simulink model "Rod_end_v7c"  (R2023a)
settings: Solver=ode1be  StartTime=0.0  StopTime=3  FixedStep=1e-6  MaxStep=1e-5  RelTol=1e-3
values from neighbouring files (symbols this model uses):
  A1_la = 5.710000e-003    (= 0.00571)    [C1_Actuator_1_Data.m]
  A2_la = 5.710000e-003    (= 0.00571)    [C1_Actuator_1_Data.m]
  a_jetpipe_area = 0    [B2_Main_file_Double_Active_Standby_System.m]
  A_svfb = 79.12.*1E-9.*sqrt(pi)    [B2_Main_file_Double_Active_Standby_System.m]
  a_svfb0_1 = 1E-3    (= 0.001)    [B2_Main_file_Double_Active_Standby_System.m]
  a_svfb0_2 = 0    [B2_Main_file_Double_Active_Standby_System.m]
  Afl_sv = dfl_sv^2*pi/4    (= 2.01519637574e-09)    [C1_Actuator_1_Data.m]
  Ag_sv = 18e-6    (= 1.8e-05)    [C1_Actuator_1_Data.m]
  air_gap0_1 = 0    [B2_Main_file_Double_Active_Standby_System.m]
  air_gap_fault_time = 10000    [B2_Main_file_Double_Active_Standby_System.m]
  Alpha_p0 = eta-acos((L^2+t^2-s^2)/(2*L*t))    [Parametri_rod_end.m]
  Asp_sv = 1.35e-5    (= 1.35e-05)    [C1_Actuator_1_Data.m]
  B0_sv = 0.460    (= 0.46)    [C1_Actuator_1_Data.m]
  b_airgap = 0.3    [B2_Main_file_Double_Active_Standby_System.m]
  b_fbspring = 2E-3    (= 0.002)    [B2_Main_file_Double_Active_Standby_System.m]
  b_max = 0*0.0001    (= 0)    [C1_Actuator_1_Data.m]
  beta = 800000000    [D4_Fluid.m]    (also in Rapporto_di_trasmissione.m = acos((L-t.*cos(alpha))./s))
  Beta0 = acos((L-t*cos(Alpha0))/s)    [Parametri_rod_end.m]
  beta_LVDT = 0    [aggiunte.m]
  bf_sv = 0.45    [C1_Actuator_1_Data.m]
  bsp_sv = 0.25    [C1_Actuator_1_Data.m]
  c = 55    [Parametri_rod_end.m]
  C_svfb = 1    [B2_Main_file_Double_Active_Standby_System.m]
  Cdmax_sv = 0.7392    [C1_Actuator_1_Data.m]
  Cdmin_sv = 0.6428    [C1_Actuator_1_Data.m]
  CLa = 900000    [aggiunte.m]
  Csa_la = 0.02*sqrt(Ksa_la*Meq_la)    [C1_Actuator_1_Data.m]
  Damping = 1e3    (= 1000)    [Parametri_rod_end.m]
  Damping_rot = 100    [Parametri_rod_end.m]
  Del_on = 1    [B2_Main_file_Double_Active_Standby_System.m]
  demag0_1 = 0    [B2_Main_file_Double_Active_Standby_System.m]
  dfl_sv = 5.0654e-5    (= 5.0654e-05)    [C1_Actuator_1_Data.m]
  dt_sim = 1e-5    (= 1e-05)    [B2_Main_file_Double_Active_Standby_System.m]
  enable_jetpipe_distorsion = 0    [B2_Main_file_Double_Active_Standby_System.m]
  eta = deg2rad(15)    [Parametri_rod_end.m]
  F_att_sv = 4    [C1_Actuator_1_Data.m]
  FH = FH+0.175*pi*Dd_se(ii)*(-0.884+0.0206*Hs_se(ii)-0.0001*(Hs_se(ii))^2)*Tw_se(ii)    [D2_Data_seal.m]
  first_cycle = 0    [B2_Main_file_Double_Active_Standby_System.m]
  flight_hours = 8    [B2_Main_file_Double_Active_Standby_System.m]
  g = 9.81    [Parametri_rod_end.m]
  g_sv = G_sv/l0_sv    (= 0)    [C1_Actuator_1_Data.m]
  Gamma_la = 1.667e4    (= 16670)    [C1_Actuator_1_Data.m]
  gap_ms = 0    [C1_Actuator_1_Data.m]
  Gq_sv = 0.069    [C1_Actuator_1_Data.m]
  Gust_stiffness_jetpipe = 1e8    (= 100000000)    [B2_Main_file_Double_Active_Standby_System.m]
  Gust_threshold = 10000    [B2_Main_file_Double_Active_Standby_System.m]
  h_fbspring = 1E-3    (= 0.001)    [B2_Main_file_Double_Active_Standby_System.m]
  h_sv = H_sv/l0_sv    (= 0)    [C1_Actuator_1_Data.m]
  hr_sv = 6e-6    (= 6e-06)    [C1_Actuator_1_Data.m]
  hyd_fluid_repl = 20    [B2_Main_file_Double_Active_Standby_System.m]
  I = 2.3    [Parametri_rod_end.m]    (also in Rapporto_di_trasmissione.m)
  imax_sv = 8e-3    (= 0.008)    [C1_Actuator_1_Data.m]
  Initial_condition = [0;0;0.000]    [Parametri_rod_end.m]
  Ixx_out = 0.0000321    (= 3.21e-05)    [Parametri_rod_end.m]
  Iyy_in = 0.0000008    (= 8e-07)    [Parametri_rod_end.m]
  Iyy_out = 0.0000035    (= 3.5e-06)    [Parametri_rod_end.m]
  Izz_in = 0.00000011    (= 1.1e-07)    [Parametri_rod_end.m]
  Izz_out = 0.0000337    (= 3.37e-05)    [Parametri_rod_end.m]
  Ja_sv = 1.0575e-5    (= 1.0575e-05)    [C1_Actuator_1_Data.m]
  jetpipe_initialpos = 0    [B2_Main_file_Double_Active_Standby_System.m]
  jetpipe_passage_area = 1    [B2_Main_file_Double_Active_Standby_System.m]
  k = 4/(3*pi*(sigma_j+sigma_k))*((R_in*R_out)/(R_in+R_out))^0.5    (= 15092124693.8)    [Parametri_rod_end.m]
  k_airgap = 0.5/100*0.01    (= 5e-05)    [B2_Main_file_Double_Active_Standby_System.m]
  k_c0_jetpipe_area = 0*1e-1    (= 0)    [B2_Main_file_Double_Active_Standby_System.m]
  k_sv = mup_sv*Vp_sv/(2*B0_sv*l0_sv)-1    (= 16.0383594613)    [C1_Actuator_1_Data.m]
  Kf_sv = 301.6    [C1_Actuator_1_Data.m]
  KFPi = zeros(m,1)    [D2_Data_seal.m]
  Kli1 = 0    [C1_Actuator_1_Data.m]
  Kli2 = 0    [C1_Actuator_1_Data.m]
  Ksa_la = 12480000    [C1_Actuator_1_Data.m]
  Kw_sv = 14.5    [C1_Actuator_1_Data.m]
  L = 0.37    [Parametri_rod_end.m]    (also in Rapporto_di_trasmissione.m = l+delta_l)
  l0_sv = 0.5e-3    (= 0.0005)    [C1_Actuator_1_Data.m]
  L_c = imax_sv    (= 0.008)    [C1_Actuator_1_Data.m]
  L_la1 = 0.059900    (= 0.0599)    [C1_Actuator_1_Data.m]
  L_la2 = 0.084800    (= 0.0848)    [C1_Actuator_1_Data.m]
  la_sv = 41e-3    (= 0.041)    [C1_Actuator_1_Data.m]
  lambda_LVDT = 0*0.005*1.5    (= 0)    [aggiunte.m]
  lf = 0.025    [C1_Actuator_1_Data.m]    (also in C2_Actuator_2_Data.m)
  LVDTsize0 = 1    [aggiunte.m]
  m_in = 0.0215    [Parametri_rod_end.m]
  m_out = 0.1    [Parametri_rod_end.m]
  m_thermal = 0    [B2_Main_file_Double_Active_Standby_System.m]
  Mcyl_la = 30.425550    (= 30.42555)    [C1_Actuator_1_Data.m]
  Mrod_la = 11.313490    (= 11.31349)    [C1_Actuator_1_Data.m]
  msp_sv = 0.005    [C1_Actuator_1_Data.m]
  mua_sv = 4*pi/1e7    (= 1.25663706144e-06)    [C1_Actuator_1_Data.m]
  mup_sv = 1.1*4*pi/1e7    (= 1.38230076758e-06)    [C1_Actuator_1_Data.m]
  n1_sv = 1140    [C1_Actuator_1_Data.m]
  n2_sv = 1140    [C1_Actuator_1_Data.m]
  n_svfb = 3    [B2_Main_file_Double_Active_Standby_System.m]
  null_shift = -1+2*rand(1,1)    [B2_Main_file_Double_Active_Standby_System.m]
  null_shift_sign = -1+((-1+2*rand(1,1))>=0)*2    [B2_Main_file_Double_Active_Standby_System.m]
  OV_R1 = 0*2.344e-05    (= 0)    [C1_Actuator_1_Data.m]
  OV_R2 = 0*2.344e-05    (= 0)    [C1_Actuator_1_Data.m]
  OV_S1 = 0*2.344e-05    (= 0)    [C1_Actuator_1_Data.m]
  OV_S2 = 0*2.344e-05    (= 0)    [C1_Actuator_1_Data.m]
  P01_la = Pmean-DP_eq    [C1_Actuator_1_Data.m]
  P02_la = Pmean+DP_eq    [C1_Actuator_1_Data.m]
  perc_passage_area0_1 = 0    [B2_Main_file_Double_Active_Standby_System.m]
  Pocl_A = 0    [C1_Actuator_1_Data.m]
  Pocl_B = 0    [C1_Actuator_1_Data.m]
  Pr = 600000    [B2_Main_file_Double_Active_Standby_System.m]
  Ps = 35000000    [B2_Main_file_Double_Active_Standby_System.m]
  R_in = 0.019    [Parametri_rod_end.m]
  R_out = 0.0195    [Parametri_rod_end.m]
  R_th1 = 0    [B2_Main_file_Double_Active_Standby_System.m]
  Remax_sv = 5000    [C1_Actuator_1_Data.m]
  Resistance = 1    [C1_Actuator_1_Data.m]
  rj_sv = 1e-6    (= 1e-06)    [C1_Actuator_1_Data.m]
  Rp02_svspring = 1014    [B2_Main_file_Double_Active_Standby_System.m]
  s = 0.11    [Parametri_rod_end.m]    (also in Rapporto_di_trasmissione.m)
  sigma_0LVDT = 0*0.01*1.5*5    (= 0)    [aggiunte.m]
  ST_AD = ceil(10000/fs_AD)/10000    [C1_Actuator_1_Data.m]
  Stiffness_rot = 1e3    (= 1000)    [Parametri_rod_end.m]
  Stifness = 1e8    (= 100000000)    [Parametri_rod_end.m]
  sv_crackON1 = 0    [B2_Main_file_Double_Active_Standby_System.m]
  sv_crackON2 = 0    [B2_Main_file_Double_Active_Standby_System.m]
  T0 = 0    [aggiunte.m]
  tau_w1 = 0    [B2_Main_file_Double_Active_Standby_System.m]
  ... (+14 more)
undefined symbols (not defined in the file or in its folder): Ixx_in, magnitude, mass, muu, Newton, R_sp_C, Raphson
libraries: simulink x16, matrix_library x12, sharedutil x2
(part 2 of 4)

== system Rod_end_v7c/Crank position/Moment ==
  M_ext : Inport
  F_ms : Inport  Port=2
  Beta : Inport  Port=3
  Alpha_p : Inport  Port=4
  Constant : Constant  Value=s
  Cos : Trigonometry  Operator=cos
  Demux : Demux  Outputs=3
  Product : Product
  Product1 : Product
  Product2 : Product
  Scope : Scope
  Sin : Trigonometry
  Subtract : Sum  Inputs=+-
  Sum : Sum
  Sum2 : Sum
  Terminator : Terminator
  M : Outport
  wires:
  Beta/1 -> Sum2/2
  Demux/1 -> Product/2
  Product/1 -> Sum/1
  Sum2/1 -> Sin/1, Cos/1
  Sum/1 -> Scope/1, Product2/2
  F_ms/1 -> Demux/1
  Product1/1 -> Sum/2
  Sin/1 -> Product/1
  Constant/1 -> Product2/1
  Demux/3 -> Terminator/1
  Cos/1 -> Product1/1
  Alpha_p/1 -> Sum2/1
  Demux/2 -> Product1/2
  Product2/1 -> Subtract/1
  Subtract/1 -> M/1
  M_ext/1 -> Subtract/2

== system Rod_end_v7c/Crank position/Rot_equilibrium ==
  note: theta_dd
  note: theta_d
  M : Inport
  M_ext : Inport  Port=2
  Angle : Inport  Port=3
  Demux : Demux  Outputs=3
  Gain : Gain  Gain=mass*g*s/3
  Gain1 : Gain  Gain=c
  Gain2 : Gain  Gain=1/I
  Integrator : Integrator
  Integrator1 : Integrator
  Sin : Trigonometry
  Sum1 : Sum  Inputs=++--
  Terminator : Terminator
  Terminator1 : Terminator
  Theta : Outport
  Theta_d : Outport  Port=2
  wires:
  Angle/1 -> Sin/1
  Sum1/1 -> Gain2/1
  Gain1/1 -> Sum1/4
  Gain2/1 -> Integrator/1
  Integrator/1 -> Integrator1/1, Theta_d/1, Gain1/1
  Gain/1 -> Sum1/3
  M/1 -> Sum1/1
  Integrator1/1 -> Theta/1
  Demux/3 -> Sum1/2
  Sin/1 -> Gain/1
  M_ext/1 -> Demux/1
  Demux/2 -> Terminator/1
  Demux/1 -> Terminator1/1

== system Rod_end_v7c/Crank position/Trigonometry for V_sup ==
  Theta_d : Inport
  Sin : Inport  Port=2
  Cos : Inport  Port=3
  Constant13 : Constant  Value=s
  Constant14 : Constant  Value=0
  Mux3 : Mux  Inputs=3
  Product12 : Product
  Product13 : Product
  Product14 : Product
  V_sup : Outport
  wires:
  Theta_d/1 -> Product12/1
  Product13/1 -> Mux3/1
  Product12/1 -> Product14/2, Product13/2
  Mux3/1 -> V_sup/1
  Constant14/1 -> Mux3/3
  Product14/1 -> Mux3/2
  Constant13/1 -> Product12/2
  Sin/1 -> Product14/1
  Cos/1 -> Product13/1

== system Rod_end_v7c/Crank position/Trigonometry for x_sup ==
  Theta : Inport
  Constant{8..11} (4 alike) : Constant  Value=s
  Constant12 : Constant  Value=0
  Constant7 : Constant  Value=pi/2-Beta0+Alpha_p0
  Cos2 : Trigonometry  Operator=cos
  Cos3 : Trigonometry  Operator=cos
  Mux2 : Mux  Inputs=3
  Product{8..11} (4 alike) : Product
  Sin2 : Trigonometry
  Sin3 : Trigonometry
  Subtract1 : Sum  Inputs=+-
  Subtract2 : Sum  Inputs=-+
  Sum3 : Sum
  X_sup : Outport
  Sin_angle+theta : Outport  Port=2
  Cos_angle+theta : Outport  Port=3
  wires:
  Sin3/1 -> Product9/2
  Sin2/1 -> Sin_angle+theta/1, Product8/2
  Cos2/1 -> Cos_angle+theta/1, Product10/2
  Product9/1 -> Subtract1/2
  Constant11/1 -> Product11/1
  Constant7/1 -> Cos3/1, Sin3/1, Sum3/2
  Product10/1 -> Subtract2/1
  Cos3/1 -> Product11/2
  Product11/1 -> Subtract2/2
  Constant10/1 -> Product10/1
  Constant8/1 -> Product8/1
  Subtract2/1 -> Mux2/2
  Constant12/1 -> Mux2/3
  Subtract1/1 -> Mux2/1
  Sum3/1 -> Cos2/1, Sin2/1
  Mux2/1 -> X_sup/1
  Product8/1 -> Subtract1/1
  Constant9/1 -> Product9/1
  Theta/1 -> Sum3/1

== system Rod_end_v7c/Molla attuatore/Linear component ==
  X_att : Inport
  V_att : Inport  Port=2
  Pos_out : Inport  Port=3
  Vel_out : Inport  Port=4
  Constant : Constant  Value=Stifness
  Constant1 : Constant  Value=Damping
  Constant2 : Constant  Value=Initial_condition
  Product : Product
  Product1 : Product
  Sum : Sum  Inputs=+--
  Sum1 : Sum  Inputs=+-
  Sum2 : Sum  Inputs=--
  F_ma : Outport
  wires:
  V_att/1 -> Sum1/2
  Constant1/1 -> Product1/2
  Sum/1 -> Product/2
  Sum1/1 -> Product1/1
  X_att/1 -> Sum/2
  Product1/1 -> Sum2/2
  Constant2/1 -> Sum/3
  Pos_out/1 -> Sum/1
  Product/1 -> Sum2/1
  Constant/1 -> Product/1
  Vel_out/1 -> Sum1/1
  Sum2/1 -> F_ma/1

== system Rod_end_v7c/Molla attuatore/Rotational  component ==
  Rot_matrix_out : Inport
  Alpha_p : Inport  Port=2
  Rot_out : Inport  Port=3
  Alpha_p_d : Inport  Port=4
  Constant : Constant  Value=Alpha_p0
  Constant{1..2,5..6} (4 alike) : Constant  Value=0
  Constant3 : Constant  Value=Stiffness_rot
  Constant4 : Constant  Value=Damping_rot
  Mux : Mux  Inputs=3
  Mux1 : Mux  Inputs=3
  Product : Product
  Product2 : Product
  Product5 : Product
  Scope6 : Scope
  Subsystem : Subsystem
  Subtract : Sum  Inputs=+-
  Subtract1 : Sum  Inputs=+-
  Subtract2 : Sum  Inputs=+-
  Sum3 : Sum
  To Workspace : ToWorkspace  VariableName=M_ext_out  SampleTime=-1
  M_ext : Outport
  wires:
  Constant5/1 -> Mux/2
  Constant3/1 -> Product/2
  Constant6/1 -> Mux/1
  Mux/1 -> Scope6/1, Subtract/2
  Product5/1 -> Sum3/2
  Constant4/1 -> Product5/2
  Subsystem/1(Angle) -> Product2/1
  Rot_matrix_out/1 -> Subsystem/1(Rot_matrix)
  Subsystem/2(Unit vector) -> Product2/2
  Product2/1 -> Subtract/1
  Sum3/1 -> To Workspace/1, M_ext/1
  Subtract/1 -> Product/1
  Product/1 -> Sum3/1
  Alpha_p/1 -> Subtract1/1
  Constant/1 -> Subtract1/2
  Subtract1/1 -> Mux/3
  Rot_out/1 -> Subtract2/1
  Subtract2/1 -> Product5/1
  Mux1/1 -> Subtract2/2
  Alpha_p_d/1 -> Mux1/3
  Constant2/1 -> Mux1/1
  Constant1/1 -> Mux1/2

== system Rod_end_v7c/Molla superficie/Linear component ==
  Pos_in : Inport
  Vel_in : Inport  Port=2
  X_sup : Inport  Port=3
  V_sup : Inport  Port=4
  Constant : Constant  Value=Stifness
  Constant1 : Constant  Value=Damping
  Product : Product
  Product1 : Product
  Sum : Sum  Inputs=+-
  Sum1 : Sum  Inputs=+-
  Sum2 : Sum  Inputs=--
  F_ms : Outport
  wires:
  Pos_in/1 -> Sum/1
  Product1/1 -> Sum2/2
  Sum2/1 -> F_ms/1
  Vel_in/1 -> Sum1/1
  Sum1/1 -> Product1/1
  X_sup/1 -> Sum/2
  Sum/1 -> Product/2
  Product/1 -> Sum2/1
  V_sup/1 -> Sum1/2
  Constant1/1 -> Product1/2
  Constant/1 -> Product/1

== system Rod_end_v7c/Molla superficie/Rotational component ==
  Rot_in : Inport
  Rot_matrix_IN : Inport  Port=2
  Theta : Inport  Port=3
  Theta_d : Inport  Port=4
  Constant{1..2,5..6} (4 alike) : Constant  Value=0
  Constant3 : Constant  Value=Stiffness_rot
  Constant4 : Constant  Value=Damping_rot
  Mux : Mux  Inputs=3
  Mux1 : Mux  Inputs=3
  Product : Product
  Product2 : Product
  Product5 : Product
  Scope : Scope
  Subsystem : Subsystem
  Subtract : Sum  Inputs=+-
  Subtract1 : Sum  Inputs=+-
  Sum3 : Sum
  To Workspace : ToWorkspace  VariableName=M_ext_in  SampleTime=-1
  M_ext : Outport
  wires:
  Product5/1 -> Sum3/2, Scope/1
  Product2/1 -> Subtract/1
  Constant4/1 -> Product5/2
  Constant2/1 -> Mux/1
  Subsystem/1(Angle) -> Product2/1
  Mux/1 -> Subtract/2
  Constant5/1 -> Mux/2
  Subsystem/2(Unit vector) -> Product2/2
  Sum3/1 -> To Workspace/1, M_ext/1
  Rot_matrix_IN/1 -> Subsystem/1(Rot_matrix)
  Constant3/1 -> Product/2
  Theta/1 -> Mux/3
  Subtract/1 -> Product/1
  Product/1 -> Sum3/1
  Rot_in/1 -> Subtract1/1
  Subtract1/1 -> Product5/1
  Mux1/1 -> Subtract1/2
  Theta_d/1 -> Mux1/3
  Constant1/1 -> Mux1/1
  Constant6/1 -> Mux1/2

== system Rod_end_v7c/Attuatore/Actuation System/Actuator ==
  In1 : Inport
  In3 : Inport  Port=2
  " " : Inport  Port=3
  Add1 : Sum  Inputs=+|-
  Add2 : Sum  Inputs=+|-
  Add3 : Sum  Inputs=+|-
  Chamber equation : Subsystem
  Constant : Constant  Value=beta
  Rod : Subsystem
  Sleeve : Subsystem
  To Workspace20 : ToWorkspace  VariableName=Att_X_cassetto  SampleTime=-1
  Out2 : Outport
  Out3 : Outport  Port=2
  Out1 : Outport  Port=3
  Out5 : Outport  Port=4
  wires:
  Chamber equation/1(Out3) -> Out2/1, Rod/3(In2), Sleeve/2(In2)  "P1;P2[Pa]"
  Constant/1 -> Chamber equation/3(In2)  "beta[Pa]"
  In1/1 -> Chamber equation/1(In4)
  In3/1 -> Chamber equation/2(In1)
  " "/1 -> Rod/2(In6)  "Fa_rod [N]"
  Sleeve/1(Out4) -> Add1/2  "xC[m]"
  Rod/3(Out4) -> Add1/1  "xR[m]"
  Rod/2(Out3) -> Add2/1  "xR_d[m/s]"
  Sleeve/2(Out3) -> Add2/2  "xC_d[m/s]"
  Add2/1 -> [x_d], Out1/1  "x_d[m/s]"
  Add1/1 -> Out3/1, [x]  "x[m]"
  [x_d] -> Chamber equation/4(In3)  "x_d[m/s]"
  [x] -> To Workspace20/1, Chamber equation/5(In5)  "x[m]"
  Rod/4(Out2) -> Sleeve/1(In4)
  [x_d] -> Rod/1(In1)  "x_d[m/s]"
  Add3/1 -> Out5/1  "x_dd[m/s^2]"
  Rod/1(Out1) -> Add3/1
  Sleeve/3(Out1) -> Add3/2

== system Rod_end_v7c/Attuatore/Actuation System/Servovalve ==
  In2 : Inport
  In1 : Inport  Port=2
  In3 : Inport  Port=3
  Demux : Demux  Outputs=2
  Servovalve Dynamic : Subsystem
  Spool : Subsystem
  Terminator : Terminator
  Terminator1 : Terminator
  Terminator2 : Terminator
  Out4 : Outport
  Out1 : Outport  Port=2
  tag scope: Act_spool=global
  wires:
  In1/1 -> Servovalve Dynamic/3(In4)  "icom1;2[A]"
  Servovalve Dynamic/1(Out1) -> Spool/3(In4), [Act_spool]  "xs[m]"
  [Fluid_properties_var] -> Servovalve Dynamic/4(In3), Spool/4(In6)  "ro;mu"
  Servovalve Dynamic/2(Out2) -> Terminator2/1
  [Supply_pressure_var] -> Servovalve Dynamic/1(In1), Spool/1(In1)  "Ps[Pa]"
  [Return_pressure_var] -> Spool/2(In5), Servovalve Dynamic/2(In2)  "Pr[Pa]"
  Spool/3(Out1) -> Out4/1  "Q1[m3/s]"
  Spool/4(Out3) -> Out1/1  "Q2[m3/s]"
  Spool/1(Out2) -> Terminator/1  "Qsup[m3/s]"
  Spool/2(Out4) -> Terminator1/1  "Qret[m3/s]"
  In2/1 -> Demux/1
  Demux/1 -> Spool/5(In2)  "P1_sb[Pa]"
  Demux/2 -> Spool/6(In3)  "P2_sb[Pa]"
  In3/1 -> Spool/7(In7)

== system Rod_end_v7c/Attuatore/Controller Actuator1/Null shift ==
  In2 : Inport
  A2[m2]1 : Gain  Gain=5/300
  A2[m2]4 : Gain  Gain=3/500
  Abs1 : Abs  SaturateOnIntegerOverflow=off
  Abs2 : Abs  SaturateOnIntegerOverflow=off
  Add1 : Sum  Inputs=+|-
  Add2 : Sum  Inputs=+|+
  Add3 : Sum  Inputs=+|-
  Constant1 : Constant  Value=Pr
  Constant2 : Constant  Value=null_shift_sign
  Constant3 : Constant  Value=20
  Constant4 : Constant  Value=null_shift
  From File2 : FromFile  FileName=E9_return_pressure.mat  SampleTime=dt_sim
  From File3 : FromFile  FileName=E10_temperature.mat  SampleTime=dt_sim
  Product1 : Product  Inputs=**/*  SaturateOnIntegerOverflow=on  OutDataTypeStr=Inherit: Same as first input
  Product2 : Product  Inputs=**/*  SaturateOnIntegerOverflow=on  OutDataTypeStr=Inherit: Same as first input
  Out2 : Outport
  wires:
  From File2/1 -> Add3/1
  Constant1/1 -> Add3/2, Product1/3
  Add3/1 -> Product1/2
  Constant2/1 -> Product1/4
  Product1/1 -> A2[m2]4/1
  In2/1 -> Abs2/1
  From File3/1 -> Add1/1
  Constant3/1 -> Add1/2, Product2/3
  Add1/1 -> Abs1/1
  Constant4/1 -> Product2/4
  Abs1/1 -> Product2/2
  Product2/1 -> A2[m2]1/1
  A2[m2]1/1 -> Add2/2
  A2[m2]4/1 -> Add2/1
  Add2/1 -> Out2/1  "Current shift [A]"
  Abs2/1 -> Product1/1, Product2/1

== system Rod_end_v7c/Contatto/Damping component/Magnitude2 ==
  vect : Inport
  Add2 : Sum  Inputs=+++
  Demux : Demux  Outputs=3
  Math Function : Math  Operator=square  SignedPower=on
  Math Function1 : Math  Operator=square  SignedPower=on
  Math Function2 : Math  Operator=square  SignedPower=on
  Sqrt : Sqrt
  mag : Outport  VectorParamsAs1DForOutWhenUnconnected=off
  wires:
  vect/1 -> Demux/1
  Add2/1 -> Sqrt/1
  Math Function2/1 -> Add2/3
  Demux/1 -> Math Function/1
  Math Function1/1 -> Add2/2
  Math Function/1 -> Add2/1
  Demux/3 -> Math Function2/1
  Demux/2 -> Math Function1/1
  Sqrt/1 -> mag/1

== system Rod_end_v7c/Contatto/Damping component/Subsystem1 ==
  note: Damping
  note: mu
  Delta_n : Inport
  Delta_d : Inport  Port=2
  Fc : Inport  Port=3
  Fcn : Fcn  Expr=(3*k*(1-e^2))/(4*u)
  Product : Product
  Subsystem : Subsystem
  To Workspace : ToWorkspace  VariableName=mu  SampleTime=-1
  D : Outport
  wires:
  Fc/1 -> Subsystem/1(Fc)
  Delta_d/1 -> Subsystem/2(Delta_d)
  Subsystem/1(Delta_d0) -> Fcn/1
  Fcn/1 -> To Workspace/1, Product/2
  Delta_n/1 -> Product/1
  Product/1 -> D/1

== system Rod_end_v7c/Contatto/Subsystem/Magnitude ==
  vect : Inport
  Add2 : Sum  Inputs=+++
  Demux : Demux  Outputs=3
  Math Function : Math  Operator=square  SignedPower=on
  Math Function1 : Math  Operator=square  SignedPower=on
  Math Function2 : Math  Operator=square  SignedPower=on
  Sqrt : Sqrt
  mag : Outport  VectorParamsAs1DForOutWhenUnconnected=off
  wires:
  vect/1 -> Demux/1
  Add2/1 -> Sqrt/1
  Math Function2/1 -> Add2/3
  Demux/1 -> Math Function/1
  Math Function1/1 -> Add2/2
  Math Function/1 -> Add2/1
  Demux/3 -> Math Function2/1
  Demux/2 -> Math Function1/1
  Sqrt/1 -> mag/1

== system Rod_end_v7c/Contatto/Subsystem1/Magnitude1 ==
  vect : Inport
  Add2 : Sum  Inputs=+++
  Demux : Demux  Outputs=3
  Math Function : Math  Operator=square  SignedPower=on
  Math Function1 : Math  Operator=square  SignedPower=on
  Math Function2 : Math  Operator=square  SignedPower=on
  Sqrt : Sqrt
  mag : Outport  VectorParamsAs1DForOutWhenUnconnected=off
  wires:
  vect/1 -> Demux/1
  Add2/1 -> Sqrt/1
  Math Function2/1 -> Add2/3
  Demux/1 -> Math Function/1
  Math Function1/1 -> Add2/2
  Math Function/1 -> Add2/1
  Demux/3 -> Math Function2/1
  Demux/2 -> Math Function1/1
  Sqrt/1 -> mag/1

== system Rod_end_v7c/Molla attuatore/Rotational  component/Subsystem ==
  Rot_matrix : Inport
  Constant : Constant
  Constant1 : Constant
  Cos : Trigonometry  Operator=acos
  Divide : Product  Inputs=/*
  Gain : Gain  Gain=1/2
  Gain1 : Gain  Gain=1/2
  Mux : Mux  Inputs=3
  Selector : Selector  NumberOfDimensions=2  InputPortWidth=3  IndexOptions=Index vector (dialog),Index vector (dialog)  Indices=1,1  OutputSizes=1,1
  Selector1 : Selector  NumberOfDimensions=2  InputPortWidth=3  IndexOptions=Index vector (dialog),Index vector (dialog)  Indices=2,2  OutputSizes=1,1
  Selector2 : Selector  NumberOfDimensions=2  InputPortWidth=3  IndexOptions=Index vector (dialog),Index vector (dialog)  Indices=3,3  OutputSizes=1,1
  Selector3 : Selector  NumberOfDimensions=2  InputPortWidth=3  IndexOptions=Index vector (dialog),Index vector (dialog)  Indices=2,3  OutputSizes=1,1
  Selector4 : Selector  NumberOfDimensions=2  InputPortWidth=3  IndexOptions=Index vector (dialog),Index vector (dialog)  Indices=3,2  OutputSizes=1,1
  Selector5 : Selector  NumberOfDimensions=2  InputPortWidth=3  IndexOptions=Index vector (dialog),Index vector (dialog)  Indices=1,3  OutputSizes=1,1
  Selector6 : Selector  NumberOfDimensions=2  InputPortWidth=3  IndexOptions=Index vector (dialog),Index vector (dialog)  Indices=3,1  OutputSizes=1,1
  Selector8 : Selector  NumberOfDimensions=2  InputPortWidth=3  IndexOptions=Index vector (dialog),Index vector (dialog)  Indices=2,1  OutputSizes=1,1
  Selector9 : Selector  NumberOfDimensions=2  InputPortWidth=3  IndexOptions=Index vector (dialog),Index vector (dialog)  Indices=1,2  OutputSizes=1,1
  Sin : Trigonometry
  Subtract : Sum  Inputs=+-
  Subtract1 : Sum  Inputs=+-
  Subtract2 : Sum  Inputs=+-
  Sum : Sum  Inputs=+++-
  Switch : Switch  Criteria=u2 ~= 0  SaturateOnIntegerOverflow=off  InputSameDT=off
  Angle : Outport
  Unit vector : Outport  Port=2
  wires:
  Selector1/1 -> Sum/2
  Selector2/1 -> Sum/3
  Selector/1 -> Sum/1
  Constant/1 -> Sum/4
  Sum/1 -> Gain/1
  Gain/1 -> Cos/1
  Cos/1 -> Angle/1, Sin/1
  Selector3/1 -> Subtract/1
  Selector4/1 -> Subtract/2
  Selector6/1 -> Subtract1/1
  Selector5/1 -> Subtract1/2
  Selector9/1 -> Subtract2/1
  Selector8/1 -> Subtract2/2
  Subtract1/1 -> Mux/2
  Subtract2/1 -> Mux/3
  Subtract/1 -> Mux/1
  Mux/1 -> Gain1/1
  Gain1/1 -> Divide/2
  Sin/1 -> Switch/1, Switch/2
  Divide/1 -> Unit vector/1
  Rot_matrix/1 -> Selector3/1, Selector8/1, Selector9/1, Selector5/1, Selector6/1, Selector4/1, Selector2/1, Selector1/1, Selector/1
  Constant1/1 -> Switch/3
  Switch/1 -> Divide/1

== system Rod_end_v7c/Molla superficie/Rotational component/Subsystem ==
  Rot_matrix : Inport
  Constant : Constant
  Constant1 : Constant
  Cos : Trigonometry  Operator=acos
  Divide : Product  Inputs=/*
  Gain : Gain  Gain=1/2
  Gain1 : Gain  Gain=1/2
  Mux : Mux  Inputs=3
  Selector : Selector  NumberOfDimensions=2  InputPortWidth=3  IndexOptions=Index vector (dialog),Index vector (dialog)  Indices=1,1  OutputSizes=1,1
  Selector1 : Selector  NumberOfDimensions=2  InputPortWidth=3  IndexOptions=Index vector (dialog),Index vector (dialog)  Indices=2,2  OutputSizes=1,1
  Selector2 : Selector  NumberOfDimensions=2  InputPortWidth=3  IndexOptions=Index vector (dialog),Index vector (dialog)  Indices=3,3  OutputSizes=1,1
  Selector3 : Selector  NumberOfDimensions=2  InputPortWidth=3  IndexOptions=Index vector (dialog),Index vector (dialog)  Indices=2,3  OutputSizes=1,1
  Selector4 : Selector  NumberOfDimensions=2  InputPortWidth=3  IndexOptions=Index vector (dialog),Index vector (dialog)  Indices=3,2  OutputSizes=1,1
  Selector5 : Selector  NumberOfDimensions=2  InputPortWidth=3  IndexOptions=Index vector (dialog),Index vector (dialog)  Indices=1,3  OutputSizes=1,1
  Selector6 : Selector  NumberOfDimensions=2  InputPortWidth=3  IndexOptions=Index vector (dialog),Index vector (dialog)  Indices=3,1  OutputSizes=1,1
  Selector8 : Selector  NumberOfDimensions=2  InputPortWidth=3  IndexOptions=Index vector (dialog),Index vector (dialog)  Indices=2,1  OutputSizes=1,1
  Selector9 : Selector  NumberOfDimensions=2  InputPortWidth=3  IndexOptions=Index vector (dialog),Index vector (dialog)  Indices=1,2  OutputSizes=1,1
  Sin : Trigonometry
  Subtract : Sum  Inputs=+-
  Subtract1 : Sum  Inputs=+-
  Subtract2 : Sum  Inputs=+-
  Sum : Sum  Inputs=+++-
  Switch : Switch  Criteria=u2 ~= 0  SaturateOnIntegerOverflow=off  InputSameDT=off
  Angle : Outport
  Unit vector : Outport  Port=2
  wires:
  Selector1/1 -> Sum/2
  Selector2/1 -> Sum/3
  Selector/1 -> Sum/1
  Constant/1 -> Sum/4
  Sum/1 -> Gain/1
  Gain/1 -> Cos/1
  Cos/1 -> Angle/1, Sin/1
  Selector3/1 -> Subtract/1
  Selector4/1 -> Subtract/2
  Selector6/1 -> Subtract1/1
  Selector5/1 -> Subtract1/2
  Selector9/1 -> Subtract2/1
  Selector8/1 -> Subtract2/2
  Subtract1/1 -> Mux/2
  Subtract2/1 -> Mux/3
  Subtract/1 -> Mux/1
  Mux/1 -> Gain1/1
  Gain1/1 -> Divide/2
  Sin/1 -> Switch/1, Switch/2
  Divide/1 -> Unit vector/1
  Rot_matrix/1 -> Selector3/1, Selector8/1, Selector9/1, Selector5/1, Selector6/1, Selector4/1, Selector2/1, Selector1/1, Selector/1
  Constant1/1 -> Switch/3
  Switch/1 -> Divide/1

== system Rod_end_v7c/Attuatore/Actuation System/Actuator/Chamber equation ==
  note: Q2_fb[m3/s]
  In4 : Inport
  In1 : Inport  Port=2
  In2 : Inport  Port=3
  In3 : Inport  Port=4
  In5 : Inport  Port=5
  Add : Sum  Inputs=+|-
  Chamber 1 : Subsystem
  Chamber 2 : Subsystem
  External leakage 1 : Fcn  Expr=Kli1*u(1)+Kli2*sqrt(abs(u(1)))
  External leakage 2 : Fcn  Expr=Kli1*u(1)+Kli2*sqrt(abs(u(1)))
  Internal leakage : Subsystem
  Mux : Mux  Inputs=2
  Out3 : Outport
  wires:
  In4/1 -> Chamber 1/1(In1)  "Q1_fb[m3/s]"
  External leakage 1/1 -> Chamber 1/6(In2)  "Qle1[m3/s]"
  Internal leakage/1(Out1) -> Chamber 1/5(In3), Chamber 2/2(In3)  "Qli[m3/s]"
  Add/1 -> Internal leakage/1(In6)  "DP[Pa]"
  Chamber 1/1(Out1) -> External leakage 1/1, Add/1, Mux/1  "P1[Pa]"
  Chamber 2/1(Out1) -> External leakage 2/1, Add/2, Mux/2  "P2[Pa]"
  In2/1 -> Chamber 1/2(In6), Chamber 2/5(In6)  "beta[Pa]"
  In3/1 -> Chamber 1/3(In5), Chamber 2/4(In5)  "x_d[m/s]"
  In5/1 -> Chamber 1/4(In4), Chamber 2/3(In4)  "x[m]"
  Mux/1 -> Out3/1  "P1;P2[Pa]"
  In1/1 -> Chamber 2/6(In1)
  External leakage 2/1 -> Chamber 2/1(In2)  "Qle2[m3/s]"

== system Rod_end_v7c/Attuatore/Actuation System/Actuator/Rod ==
  In1 : Inport
  In6 : Inport  Port=2
  In2 : Inport  Port=3
  1/Mrod[1/kg] : Gain  Gain=1/Mrod_la
  A1[m2] : Gain  Gain=A1_la
  A2[m2] : Gain  Gain=A2_la
  Add1 : Sum  Inputs=+|-|+
  Demux : Demux  Outputs=2
  Double Integrator : Subsystem
  Friction1 : Subsystem
  Gamma[Ns/m] : Gain  Gain=Gamma_la
  To Workspace20 : ToWorkspace  VariableName=Att_F_attrito  SampleTime=-1
  Out1 : Outport
  Out3 : Outport  Port=2
  Out4 : Outport  Port=3
  Out2 : Outport  Port=4
  wires:
  Add1/1 -> Friction1/2(In1)  "Fact[N]"
  Demux/1 -> A1[m2]/1  "P1[Pa]"
  Demux/2 -> A2[m2]/1  "P2[Pa]"
  In2/1 -> Demux/1, Friction1/1(In3)  "P1;P2[Pa]"
  Friction1/2(Out1) -> 1/Mrod[1/kg]/1
  1/Mrod[1/kg]/1 -> Out1/1, Double Integrator/1(In1)  "xR_dd[m2/s]"
  Double Integrator/2(Out2) -> Out3/1, Friction1/4(In2)  "xR_d[m/s]"
  A1[m2]/1 -> Add1/1
  A2[m2]/1 -> Add1/2
  Double Integrator/1(Out1) -> Out4/1  "xR[m]"
  In1/1 -> Gamma[Ns/m]/1  "x_d[m/s]"
  Friction1/1(Out2) -> To Workspace20/1, Out2/1  "Ffrict[N]"
  Friction1/3(Out3) -> Double Integrator/2(In2)
  Double Integrator/3(Out3) -> Friction1/5(In4)
  In6/1 -> Add1/3  "Fext[N]"
  Gamma[Ns/m]/1 -> Friction1/3(In5)

== system Rod_end_v7c/Attuatore/Actuation System/Actuator/Sleeve ==
  In4 : Inport
  In2 : Inport  Port=2
  1/Mcyl[1/kg] : Gain  Gain=1/Mcyl_la
  A1[m2] : Gain  Gain=A1_la
  A2[m2] : Gain  Gain=A2_la
  Add1 : Sum  Inputs=-|+|-
  Add3 : Sum  Inputs=+|-
  Backlash : Subsystem
  Demux : Demux  Outputs=2
  Integrator : Integrator
  Integrator1 : Integrator
  Out4 : Outport
  Out3 : Outport  Port=2
  Out1 : Outport  Port=3
  wires:
  Demux/1 -> A1[m2]/1  "P1[Pa]"
  Demux/2 -> A2[m2]/1  "P2[Pa]"
  In2/1 -> Demux/1  "P1;P2[Pa]"
  A1[m2]/1 -> Add1/1
  A2[m2]/1 -> Add1/2
  Integrator/1 -> Integrator1/1, Out3/1, Backlash/1(In2)  "xC_d[m/s]"
  Integrator1/1 -> Out4/1, Backlash/2(In1)  "xC [m]"
  In4/1 -> Add1/3  "Ffrict[N]"
  1/Mcyl[1/kg]/1 -> Out1/1, Integrator/1  "xC_dd [m/s^2]"
  Add1/1 -> Add3/1  "Fact[N]"
  Backlash/1(Out1) -> Add3/2  "Fext_sl[N]"
  Add3/1 -> 1/Mcyl[1/kg]/1

== system Rod_end_v7c/Attuatore/Actuation System/Servovalve/Servovalve Dynamic ==
  In1 : Inport
  In2 : Inport  Port=2
  In4 : Inport  Port=3
  In3 : Inport  Port=4
  Crack propagation : Subsystem
  First Stage Leakage : Subsystem
  Hydraulic amplifier : Subsystem
  Jet pipe dynamic : Subsystem
  Saturation2 : Saturate  UpperLimit=Ps-Pr  LowerLimit=-(Ps-Pr)
  Spool  dynamic : Subsystem
  To Workspace1 : ToWorkspace  VariableName=Att_X_flapper  SampleTime=-1
  To Workspace2 : ToWorkspace  VariableName=Att_X_spool  SampleTime=-1
  To Workspace20 : ToWorkspace  VariableName=Att_C_torque_motor  SampleTime=-1
  Torque Motor : Subsystem
  Out1 : Outport
  Out2 : Outport  Port=2
  wires:
  In4/1 -> Torque Motor/1(In4)  "icom(1;2)[A]"
  In2/1 -> First Stage Leakage/2(In2), Hydraulic amplifier/3(In3)  "Pr[Pa]"
  In1/1 -> First Stage Leakage/1(In1), Hydraulic amplifier/2(In2)  "Ps[Pa]"
  First Stage Leakage/1(Out1) -> Out2/1  "QLfs[m3/s]"
  In3/1 -> First Stage Leakage/3(In4)  "ro;mu"
  Spool  dynamic/2(Out2) -> Hydraulic amplifier/4(In1)  "dxs[m/s]"
  Spool  dynamic/1(Out1) -> To Workspace2/1, Jet pipe dynamic/1(In1), Out1/1  "xs[m]"
  Hydraulic amplifier/1(Out1) -> Saturation2/1  "dP[Pa]"
  Jet pipe dynamic/1(Out1) -> To Workspace1/1, Spool  dynamic/1(In1), Hydraulic amplifier/1(In4)  "xf[m]"
  Saturation2/1 -> Spool  dynamic/2(In4)
  Jet pipe dynamic/2(Out2) -> Torque Motor/2(In1)
  Torque Motor/1(Out1) -> Crack propagation/1(Tb [N/m]), To Workspace20/1, Jet pipe dynamic/2(In4)  "Torque [Nm]"
  Crack propagation/1(Kw_mod) -> Jet pipe dynamic/3(In2), Spool  dynamic/3(In2)
  [flight_time] -> Hydraulic amplifier/5(In5)

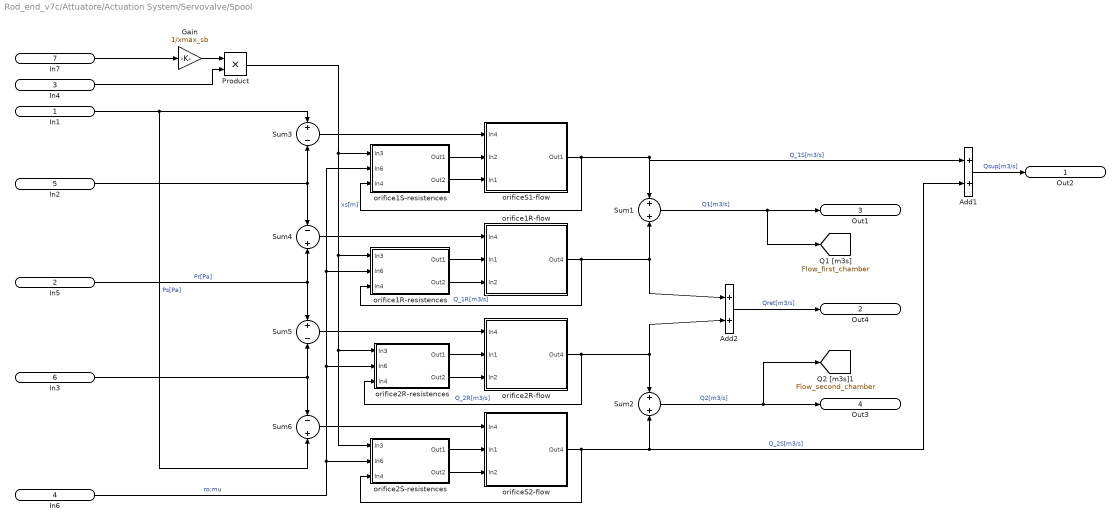
== system Rod_end_v7c/Attuatore/Actuation System/Servovalve/Spool ==
  In1 : Inport
  In5 : Inport  Port=2
  In4 : Inport  Port=3
  In6 : Inport  Port=4
  In2 : Inport  Port=5
  In3 : Inport  Port=6
  In7 : Inport  Port=7
  Add1 : Sum  Inputs=+|+
  Add2 : Sum  Inputs=+|+
  Gain : Gain  Gain=1/xmax_sb
  Product : Product  RndMeth=Zero
  Sum1 : Sum  Inputs=+|+  SaturateOnIntegerOverflow=on
  Sum2 : Sum  Inputs=+|+  SaturateOnIntegerOverflow=on
  Sum3 : Sum  Inputs=+-  SaturateOnIntegerOverflow=on
  Sum4 : Sum  Inputs=-|+  SaturateOnIntegerOverflow=on
  Sum5 : Sum  Inputs=+|-  SaturateOnIntegerOverflow=on
  Sum6 : Sum  Inputs=-+  SaturateOnIntegerOverflow=on
  orifice1R-flow : Subsystem
  orifice1R-resistences : Subsystem
  orifice1S-resistences : Subsystem
  orifice2R-flow : Subsystem
  orifice2R-resistences : Subsystem
  orifice2S-resistences : Subsystem
  orificeS1-flow : Subsystem
  orificeS2-flow : Subsystem
  Out2 : Outport
  Out4 : Outport  Port=2
  Out1 : Outport  Port=3
  Out3 : Outport  Port=4
  tag scope: Flow_first_chamber=global, Flow_second_chamber=global
  wires:
  orificeS1-flow/1(Out1) -> Sum1/1, Add1/1, orifice1S-resistences/3(In4)  "Q_1S[m3/s]"
  orifice1R-flow/1(Out4) -> Add2/1, Sum1/2, orifice1R-resistences/3(In4)  "Q_1R[m3/s]"
  Sum4/1 -> orifice1R-flow/1(In4)
  Sum3/1 -> orificeS1-flow/1(In4)
  In2/1 -> Sum4/1, Sum3/2
  In3/1 -> Sum5/2, Sum6/1
  In1/1 -> Sum6/2, Sum3/1  "Ps[Pa]"
  Sum1/1 -> Out1/1, [Flow_first_chamber]  "Q1[m3/s]"
  Sum2/1 -> Out3/1, [Flow_second_chamber]  "Q2[m3/s]"
  orifice2S-resistences/1(Out1) -> orificeS2-flow/2(In1)
  Sum5/1 -> orifice2R-flow/1(In4)
  orifice2R-flow/1(Out4) -> Add2/2, Sum2/1, orifice2R-resistences/3(In4)  "Q_2R[m3/s]"
  orifice2S-resistences/2(Out2) -> orificeS2-flow/3(In2)
  orificeS2-flow/1(Out4) -> Sum2/2, Add1/2, orifice2S-resistences/3(In4)  "Q_2S[m3/s]"
  In5/1 -> Sum5/1, Sum4/2  "Pr[Pa]"
  Add1/1 -> Out2/1  "Qsup[m3/s]"
  Add2/1 -> Out4/1  "Qret[m3/s]"
  Product/1 -> orifice1S-resistences/1(In3), orifice2R-resistences/1(In3), orifice2S-resistences/1(In3), orifice1R-resistences/1(In3)  "xs[m]"
  In6/1 -> orifice1S-resistences/2(In6), orifice1R-resistences/2(In6), orifice2R-resistences/2(In6), orifice2S-resistences/2(In6)  "ro;mu"
  orifice2R-resistences/1(Out1) -> orifice2R-flow/2(In1)
  orifice2R-resistences/2(Out2) -> orifice2R-flow/3(In2)
  Sum6/1 -> orificeS2-flow/1(In4)
  orifice1R-resistences/1(Out1) -> orifice1R-flow/2(In1)
  orifice1R-resistences/2(Out2) -> orifice1R-flow/3(In2)
  orifice1S-resistences/1(Out1) -> orificeS1-flow/2(In2)
  orifice1S-resistences/2(Out2) -> orificeS1-flow/3(In1)
  In7/1 -> Gain/1
  Gain/1 -> Product/1
  In4/1 -> Product/2

== system Rod_end_v7c/Contatto/Damping component/Subsystem1/Subsystem ==
  Fc : Inport
  Delta_d : Inport  Port=2
  Compare To Constant1 : simulink/Logic and Bit Operations/Compare To Constant  relop===  const=0  OutDataTypeStr=boolean
  Data Store Memory : DataStoreMemory  DataStoreName=Delta_d0  WriteAfterWriteMsg=warning  ShowAdditionalParam=off
  Data Store Read : DataStoreRead  DataStoreName=Delta_d0  IndexOptions=Index vector (dialog)  Indices=1  OutputSizes=1
  Data Store Write : DataStoreWrite  DataStoreName=Delta_d0  IndexOptions=Index vector (dialog)  Indices=1  OutputSizes=1
  Display{1..7} (7 alike) : Display
  Logical Operator : Logic  Operator=NOT  AllPortsSameDT=off  OutDataTypeStr=boolean
  Magnitude2 : Subsystem
  Memory : Memory
  Switch : Switch  Criteria=u2 ~= 0  SaturateOnIntegerOverflow=off  InputSameDT=off
  Delta_d0 : Outport
  wires:
  Fc/1 -> Display1/1, Magnitude2/1(vect)
  Compare To Constant1/1 -> Display2/1, Logical Operator/1
  Logical Operator/1 -> Display3/1, Memory/1
  Memory/1 -> Display7/1, Switch/2
  Switch/1 -> Delta_d0/1, Display6/1, Data Store Write/1
  Magnitude2/1(mag) -> Compare To Constant1/1
  Data Store Read/1 -> Switch/1, Display4/1
  Delta_d/1 -> Display5/1, Switch/3

== system Rod_end_v7c/Attuatore/Actuation System/Actuator/Chamber equation/Chamber 1 ==
  In1 : Inport
  In6 : Inport  Port=2
  In5 : Inport  Port=3
  In4 : Inport  Port=4
  In3 : Inport  Port=5
  In2 : Inport  Port=6
  Integrator : Integrator  InitialCondition=P01_la  LimitOutput=on  UpperSaturationLimit=Ps  LowerSaturationLimit=Pr
  Mux : Mux  Inputs=6
  chamber1 equation : Fcn  Expr=u(2)*(u(1)-u(6)-u(5)-u(3)*A1_la)/(V01_la+u(4)*A1_la)
  Out1 : Outport
  wires:
  In1/1 -> Mux/1  "Q1[m3/s]"
  In2/1 -> Mux/6  "Qle1[m3/s]"
  In3/1 -> Mux/5  "Qli[m3/s]"
  In4/1 -> Mux/4  "z[m]"
  In5/1 -> Mux/3  "z_d[m/s]"
  In6/1 -> Mux/2  "beta[Pa]"
  chamber1 equation/1 -> Integrator/1  "dP1[Pa/s]"
  Integrator/1 -> Out1/1  "P1[Pa]"
  Mux/1 -> chamber1 equation/1

== system Rod_end_v7c/Attuatore/Actuation System/Actuator/Chamber equation/Chamber 2 ==
  In2 : Inport
  In3 : Inport  Port=2
  In4 : Inport  Port=3
  In5 : Inport  Port=4
  In6 : Inport  Port=5
  In1 : Inport  Port=6
  Integrator : Integrator  InitialCondition=P02_la  LimitOutput=on  UpperSaturationLimit=Ps  LowerSaturationLimit=Pr
  Mux : Mux  Inputs=6
  chamber2 equation : Fcn  Expr=u(2)*(u(1)-u(6)+u(5)+u(3)*A2_la)/(V02_la-u(4)*A2_la)
  Out1 : Outport
  wires:
  In1/1 -> Mux/1  "Q2[m3/s]"
  Mux/1 -> chamber2 equation/1
  In2/1 -> Mux/6  "Qle2[m3/s]"
  In3/1 -> Mux/5  "Qli[m3/s]"
  In4/1 -> Mux/4  "z[m]"
  In5/1 -> Mux/3  "z_d[m/s]"
  In6/1 -> Mux/2  "beta[Pa]"
  chamber2 equation/1 -> Integrator/1  "dP2[Pa/s]"
  Integrator/1 -> Out1/1  "P2[Pa]"

== system Rod_end_v7c/Attuatore/Actuation System/Actuator/Chamber equation/Internal leakage ==
  In6 : Inport
  Internal leakage : Fcn  Expr=Kli1*u(1)+Kli2*sqrt(abs(u(1)))*u(2)
  Mux : Mux  Inputs=2
  Sign : Signum
  Out1 : Outport
  wires:
  In6/1 -> Sign/1, Mux/1  "DP[Pa]"
  Sign/1 -> Mux/2
  Mux/1 -> Internal leakage/1
  Internal leakage/1 -> Out1/1  "Qli[m3/s]"

== system Rod_end_v7c/Attuatore/Actuation System/Actuator/Rod/Double Integrator ==
  In1 : Inport
  In2 : Inport  Port=2
  Abs : Abs  SaturateOnIntegerOverflow=off
  Compare To Constant : simulink/Logic and Bit Operations/Compare To Constant  relop===  const=1  OutDataTypeStr=boolean
  Compare To Constant1 : simulink/Logic and Bit Operations/Compare To Constant  relop===  const=1  OutDataTypeStr=boolean
  Integrator : Integrator  ExternalReset=rising  ShowStatePort=on
  Integrator1 : Integrator  InitialCondition=x0_la  LimitOutput=on  UpperSaturationLimit=L_la2  LowerSaturationLimit=-L_la1  ShowSaturationPort=on
  Limit : Subsystem
  Logical Operator : Logic  Operator=OR  AllPortsSameDT=off  OutDataTypeStr=boolean
  Out1 : Outport
  Out2 : Outport  Port=2
  Out3 : Outport  Port=3
  wires:
  Integrator/1 -> Integrator1/1, Out2/1  "xR_d[m/s]"
  Integrator1/1 -> Out1/1  "xR[m]"
  Limit/1(Out2) -> Integrator/1
  Integrator1/2 -> Limit/2(In1), Abs/1  "limit xatt"
  In1/1 -> Limit/1(In2)  "xR_dd[m/s2]"
  Abs/1 -> Compare To Constant/1
  In2/1 -> Compare To Constant1/1
  Compare To Constant1/1 -> Logical Operator/1
  Compare To Constant/1 -> Logical Operator/2
  Logical Operator/1 -> Integrator/2
  Integrator/State -> Out3/1  "zero-crossing"

== system Rod_end_v7c/Attuatore/Actuation System/Actuator/Rod/Friction1 ==
  In3 : Inport
  In1 : Inport  Port=2
  In5 : Inport  Port=3
  In2 : Inport  Port=4
  In4 : Inport  Port=5
  Abs : Abs  SaturateOnIntegerOverflow=off
  Add2 : Sum  Inputs=+|-
  FP : Subsystem
  Fcoul : Fcn  Expr=((u(2))*(1+(0.5)*exp(-10*abs(u(1))))+abs(u(3)))
  Hit Crossing : HitCross  HitCrossingOffset=0.0
  MinMax : MinMax  Inputs=2
  Mux1 : Mux  Inputs=3
  Mux2 : Mux  Inputs=2
  Mux3 : Mux  Inputs=3
  Product : Product  RndMeth=Zero
  Scope1 : Scope
  Scope2 : Scope
  Scope3 : Scope
  Sign1 : Signum
  Sign3 : Signum
  Switch : Switch  Criteria=u2 > Threshold  Threshold=0.0  SaturateOnIntegerOverflow=off  InputSameDT=off
  Switch1 : Switch  Criteria=u2 > Threshold  Threshold=0.0  SaturateOnIntegerOverflow=off  InputSameDT=off
  Out2 : Outport
  Out1 : Outport  Port=2
  Out3 : Outport  Port=3
  wires:
  Fcoul/1 -> MinMax/2, Mux3/3, Switch1/3  "Fcoul[N]"
  FP/1(Out4) -> Mux1/2
  In3/1 -> FP/1(In3)  "P[Pa]"
  Mux1/1 -> Fcoul/1
  In2/1 -> Mux1/1, Sign3/1  "x_d[m/s]"
  Add2/1 -> Out1/1  "Fctr[N]"
  Abs/1 -> Mux3/2, MinMax/1
  In1/1 -> Sign1/1, Abs/1, Mux2/1, Add2/1  "Factive[N]"
  Hit Crossing/1 -> Switch1/2, Scope1/1, Out3/1, Switch/2  "reset"
  Sign1/1 -> Switch/1
  Switch/1 -> Product/1
  MinMax/1 -> Mux3/1, Switch1/1
  Product/1 -> Add2/2, Mux2/2, Out2/1  "Ffrict[N]"
  In4/1 -> Hit Crossing/1
  Switch1/1 -> Product/2
  Sign3/1 -> Switch/3
  In5/1 -> Mux1/3  "viscous friction"
  Mux2/1 -> Scope2/1
  Mux3/1 -> Scope3/1

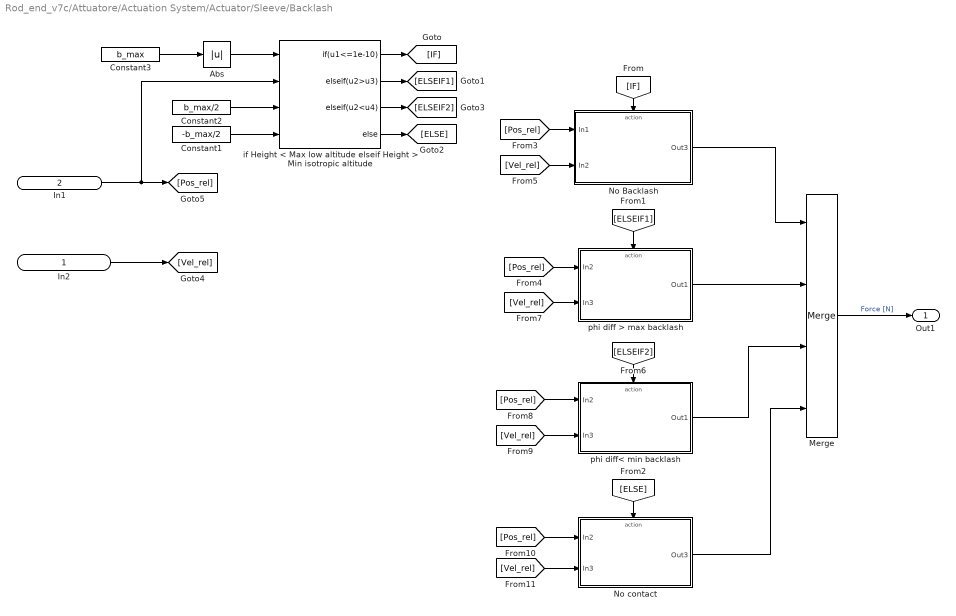
== system Rod_end_v7c/Attuatore/Actuation System/Actuator/Sleeve/Backlash ==
  In2 : Inport
  In1 : Inport  Port=2
  Abs : Abs  SaturateOnIntegerOverflow=off
  Constant1 : Constant  Value=-b_max/2
  Constant2 : Constant  Value=b_max/2
  Constant3 : Constant  Value=b_max
  Merge : Merge  Inputs=4
  No Backlash : Subsystem  TreatAsAtomicUnit=on
  No contact : Subsystem  TreatAsAtomicUnit=on
  "if Height < Max low altitude elseif Height > Min isotropic altitude " : If  NumInputs=4  IfExpression=u1<=1e-10  ElseIfExpressions=u2>u3, u2<u4
  phi diff > max backlash : Subsystem  TreatAsAtomicUnit=on
  phi diff< min backlash : Subsystem  TreatAsAtomicUnit=on
  Out1 : Outport
  wires:
  "if Height < Max low altitude elseif Height > Min isotropic altitude "/1 -> [IF]
  "if Height < Max low altitude elseif Height > Min isotropic altitude "/2 -> [ELSEIF1]
  "if Height < Max low altitude elseif Height > Min isotropic altitude "/4 -> [ELSE]
  Abs/1 -> "if Height < Max low altitude elseif Height > Min isotropic altitude "/1
  In1/1 -> [Pos_rel], "if Height < Max low altitude elseif Height > Min isotropic altitude "/2
  Constant2/1 -> "if Height < Max low altitude elseif Height > Min isotropic altitude "/3
  Constant1/1 -> "if Height < Max low altitude elseif Height > Min isotropic altitude "/4
  "if Height < Max low altitude elseif Height > Min isotropic altitude "/3 -> [ELSEIF2]
  In2/1 -> [Vel_rel]
  [Pos_rel] -> No Backlash/1(In1)
  [Vel_rel] -> No Backlash/2(In2)
  [ELSEIF1] -> phi diff > max backlash/Action
  [IF] -> No Backlash/Action
  [Vel_rel] -> phi diff > max backlash/2(In3)
  [Pos_rel] -> phi diff > max backlash/1(In2)
  [ELSEIF2] -> phi diff< min backlash/Action
  [Vel_rel] -> phi diff< min backlash/2(In3)
  [Pos_rel] -> phi diff< min backlash/1(In2)
  No Backlash/1(Out3) -> Merge/1
  phi diff > max backlash/1(Out1) -> Merge/2
  phi diff< min backlash/1(Out1) -> Merge/3
  Merge/1 -> Out1/1  "Force [N]"
  [ELSE] -> No contact/Action
  No contact/1(Out3) -> Merge/4
  [Pos_rel] -> No contact/1(In2)
  [Vel_rel] -> No contact/2(In3)
  Constant3/1 -> Abs/1

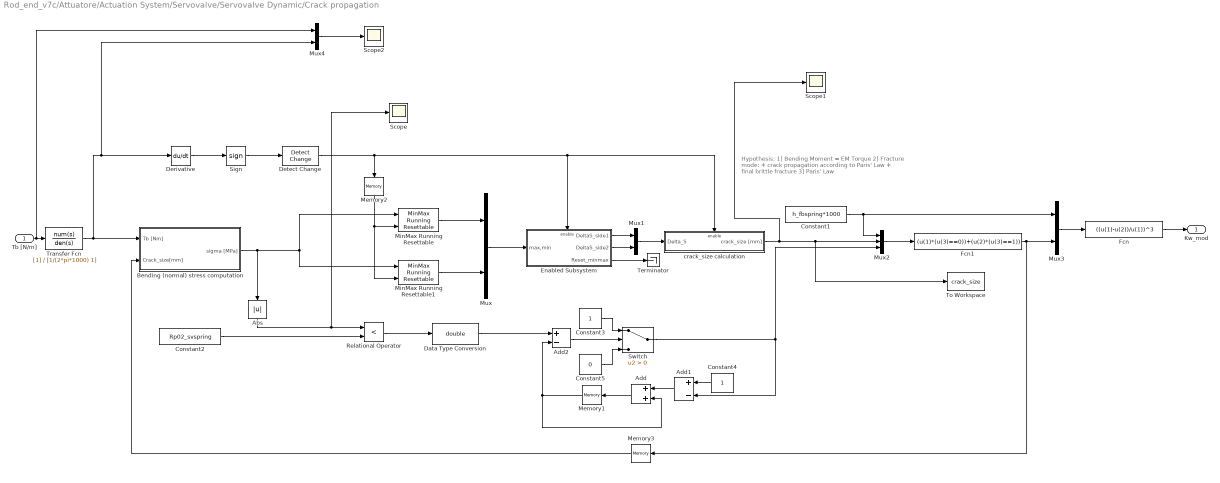
== system Rod_end_v7c/Attuatore/Actuation System/Servovalve/Servovalve Dynamic/Crack propagation ==
  note: Hypothesis:
      | 1] Bending Moment = EM Torque
      | 2] Fracture mode:
      | 		+ crack propagation according to Paris' Law
      | 		+ final brittle fracture
      | 3] Paris' Law
  Tb [N/m] : Inport
  Abs : Abs  SaturateOnIntegerOverflow=off
  Add : Sum
  Add1 : Sum  Inputs=+-
  Add2 : Sum  Inputs=+-
  Bending (normal) stress computation : Subsystem
  Constant1 : Constant  Value=h_fbspring*1000
  Constant2 : Constant  Value=Rp02_svspring
  Constant3 : Constant
  Constant4 : Constant
  Constant5 : Constant  Value=0
  Data Type Conversion : DataTypeConversion  OutDataTypeStr=double  SaturateOnIntegerOverflow=off  RndMeth=Floor
  Derivative : Derivative
  Detect Change : simulink/Logic and Bit Operations/Detect Change  vinit=0  OutDataTypeStr=uint8
  Enabled Subsystem : Subsystem  TreatAsAtomicUnit=on
  Fcn : Fcn  Expr=((u(1)-u(2))/u(1))^3
  Fcn1 : Fcn  Expr=(u(1)*(u(3)==0))+(u(2)*(u(3)==1))
  Memory1 : Memory
  Memory2 : Memory
  Memory3 : Memory
  MinMax Running Resettable : simulink/Math Operations/MinMax Running Resettable  Function=max  vinit=0.0
  MinMax Running Resettable1 : simulink/Math Operations/MinMax Running Resettable  Function=min  vinit=0.0
  Mux{,1,3..4} (4 alike) : Mux  Inputs=2
  Mux2 : Mux  Inputs=3
  Relational Operator : RelationalOperator  Operator=<  OutDataTypeStr=boolean  InputSameDT=off
  Scope : Scope
  Scope1 : Scope
  Scope2 : Scope
  Sign : Signum
  Switch : Switch  Criteria=u2 > Threshold  SaturateOnIntegerOverflow=off  InputSameDT=off
  Terminator : Terminator
  To Workspace : ToWorkspace  VariableName=crack_size  SaveFormat=Structure With Time  SampleTime=-1
  Transfer Fcn : TransferFcn  Denominator=[1/(2*pi*1000) 1]
  crack_size calculation : Subsystem
  Kw_mod : Outport
  wires:
  Memory3/1 -> Bending (normal) stress computation/2(Crack_size[mm])
  Derivative/1 -> Sign/1
  Mux/1 -> Enabled Subsystem/1(max,min)
  Bending (normal) stress computation/1(sigma [MPa]) -> MinMax Running Resettable/1, MinMax Running Resettable1/1, Abs/1
  MinMax Running Resettable/1 -> Mux/1
  MinMax Running Resettable1/1 -> Mux/2
  Enabled Subsystem/1(DeltaS_side1) -> Mux1/1
  Enabled Subsystem/2(DeltaS_side2) -> Mux1/2
  Mux1/1 -> crack_size calculation/1(Delta_S)
  crack_size calculation/1(crack_size [mm]) -> Scope1/1, To Workspace/1, Mux2/2
  Constant1/1 -> Mux2/1, Mux3/1
  Constant2/1 -> Relational Operator/2
  Relational Operator/1 -> Data Type Conversion/1
  Fcn/1 -> Kw_mod/1
  Sign/1 -> Detect Change/1
  Detect Change/1 -> Memory2/1, Enabled Subsystem/Enable, crack_size calculation/Enable
  Constant3/1 -> Switch/1
  Constant4/1 -> Add1/1
  Add/1 -> Memory1/1
  Memory1/1 -> Add2/2, Add/2
  Add1/1 -> Add/1
  Constant5/1 -> Switch/3
  Switch/1 -> Mux2/3, Add1/2
  Data Type Conversion/1 -> Add2/1
  Add2/1 -> Switch/2
  Fcn1/1 -> Mux3/2, Memory3/1
  Mux3/1 -> Fcn/1
  Memory2/1 -> MinMax Running Resettable1/2, MinMax Running Resettable/2
  Mux2/1 -> Fcn1/1
  Enabled Subsystem/3(Reset_minmax) -> Terminator/1
  Abs/1 -> Scope/1, Relational Operator/1
  Tb [N/m]/1 -> Mux4/1, Transfer Fcn/1
  Mux4/1 -> Scope2/1
  Transfer Fcn/1 -> Mux4/2, Derivative/1, Bending (normal) stress computation/1(Tb [Nm])

== system Rod_end_v7c/Attuatore/Actuation System/Servovalve/Servovalve Dynamic/First Stage Leakage ==
  In1 : Inport
  In2 : Inport  Port=2
  In4 : Inport  Port=3
  Add1 : Sum  Inputs=+|-
  Fcn : Fcn  Expr=0.22*sqrt(log(1+u(2)))*Afl_sv*sqrt(u(1))
  Memory : Memory  InitialCondition=5.74e-6
  Mux1 : Mux  Inputs=2
  Mux2 : Mux  Inputs=2
  Reynold : Fcn  Expr=u(1)*(u(3)/Afl_sv)*dfl_sv/(u(2))
  Saturation : Saturate  UpperLimit=5000  LowerLimit=0
  Out1 : Outport
  wires:
  Saturation/1 -> Mux1/2  "Re"
  In1/1 -> Add1/1  "Ps[Pa]"
  Reynold/1 -> Saturation/1  "Re"
  Mux1/1 -> Fcn/1
  Fcn/1 -> Out1/1, Memory/1  "QLfs[m3/s]"
  Add1/1 -> Mux1/1  "dP[Pa]"
  In2/1 -> Add1/2  "Pr[Pa]"
  Mux2/1 -> Reynold/1
  In4/1 -> Mux2/1  "ro;mu"
  Memory/1 -> Mux2/2  "Qlfs[m3/s]"

== system Rod_end_v7c/Attuatore/Actuation System/Servovalve/Servovalve Dynamic/Hydraulic amplifier ==
  In4 : Inport
  In2 : Inport  Port=2
  In3 : Inport  Port=3
  In1 : Inport  Port=4
  In5 : Inport  Port=5
  Add2 : Sum  Inputs=+|-
  Jetpipe area occlusion : Subsystem
  Scope3 : Scope
  Ugello A : Subsystem
  Ugello B : Subsystem
  Out1 : Outport
  wires:
  In1/1 -> Ugello A/2(In2), Ugello B/4(In2)  "dxs[m/s]"
  Add2/1 -> Out1/1  "Dp"
  Ugello B/1(PB) -> Add2/2
  Ugello A/1(PA) -> Add2/1
  In4/1 -> Ugello A/1(In4), Ugello B/5(In4)  "xf[m]"
  In2/1 -> Ugello A/3(In1), Ugello B/3(In1)
  In3/1 -> Ugello A/4(In3), Ugello B/2(In3)
  Jetpipe area occlusion/1(Out2) -> Ugello B/1(In5), Scope3/1, Ugello A/5(In5)
  In5/1 -> Jetpipe area occlusion/1(In1)

== system Rod_end_v7c/Attuatore/Actuation System/Servovalve/Servovalve Dynamic/Jet pipe dynamic ==
  In1 : Inport
  In4 : Inport  Port=2
  In2 : Inport  Port=3
  Add1 : Sum  Inputs=+|-|-|-
  Add2 : Sum  Inputs=+|+
  Dead Zone : DeadZone  LowerValue=-gap_ms/2  UpperValue=gap_ms/2
  Double Integrator : Subsystem
  Gain : Gain  Gain=1/Ja_sv
  Gain1 : Gain  Gain=Kw_sv
  Gain3 : Gain  Gain=Kf_sv
  Gain4 : Gain  Gain=bf_sv
  Gain5 : Gain  Gain=0.7
  Jetpipe distorted : Subsystem
  Mux1 : Mux  Inputs=2
  Product1 : Product  SaturateOnIntegerOverflow=on  OutDataTypeStr=Inherit: Same as first input
  Scope : Scope
  Out1 : Outport
  Out2 : Outport  Port=2
  wires:
  In4/1 -> Add1/1  "Torque [N]"
  Add1/1 -> Gain/1
  Gain/1 -> Double Integrator/1(In1)  "ddxf[m2/s]"
  Jetpipe distorted/1(Out2) -> Add2/2, Gain3/1, Out1/1, Gain5/1, Mux1/2  "xf[m]"
  Gain3/1 -> Add1/3
  Gain5/1 -> Out2/1  "xa[m]"
  Add2/1 -> Dead Zone/1
  In1/1 -> Add2/1  "xs[m]"
  Gain4/1 -> Add1/4
  Double Integrator/2(Out2) -> Gain4/1
  Dead Zone/1 -> Gain1/1
  [turbolence_on_jetpipe] -> Jetpipe distorted/1(In3)
  Double Integrator/1(Out1) -> Jetpipe distorted/2(In1), Mux1/1
  Mux1/1 -> Scope/1
  Product1/1 -> Add1/2
  In2/1 -> Product1/1  "Kw_modifier"
  Gain1/1 -> Product1/2  "Fb[Nm]"

== system Rod_end_v7c/Attuatore/Actuation System/Servovalve/Servovalve Dynamic/Spool  dynamic ==
  In1 : Inport
  In4 : Inport  Port=2
  In2 : Inport  Port=3
  Add1 : Sum  Inputs=-|+
  Add2 : Sum  Inputs=+|+
  Add3 : Sum  Inputs=+|+
  Dead Zone : DeadZone  LowerValue=-gap_ms/2  UpperValue=gap_ms/2
  Double Integrator : Subsystem
  Flow Force : Subsystem
  Friction : Subsystem
  Gain : Gain  Gain=1/msp_sv
  Gain2 : Gain  Gain=Kw_sv/lf
  Gain3 : Gain  Gain=Asp_sv
  Product1 : Product  SaturateOnIntegerOverflow=on  OutDataTypeStr=Inherit: Same as first input
  Out1 : Outport
  Out2 : Outport  Port=2
  wires:
  Gain/1 -> Double Integrator/1(In1)  "ddxs [m2/s]"
  Double Integrator/2(Out2) -> Out2/1, Friction/2(In2)  "dxs[m/s]"
  Double Integrator/1(Out1) -> Out1/1, Flow Force/1(In1), Add2/1  "xs[m]"
  In4/1 -> Gain3/1  "dP[Pa]"
  Gain3/1 -> Add1/2
  In1/1 -> Add2/2  "xf[m]"
  Add2/1 -> Dead Zone/1
  Friction/1(Out1) -> Gain/1
  Dead Zone/1 -> Gain2/1
  Add3/1 -> Friction/1(In1)  "F_res [N]"
  Add1/1 -> Add3/2  "F_res [N]"
  Friction/2(Out2) -> Double Integrator/2(In2)
  Double Integrator/3(Out3) -> Friction/3(In3)
  Flow Force/1(Ffl1+Ffl2) -> Add3/1
  Gain2/1 -> Product1/1  "Ffb[N]"
  In2/1 -> Product1/2  "Kw_modifier"
  Product1/1 -> Add1/1
